simulink model "lane_rule"  (R2016b)
settings: Solver=VariableStepAuto  StartTime=0.0  StopTime=10.0  RelTol=1e-3
libraries: robotlib x13
settings Model: Creator=shota  LastModifiedBy=shota

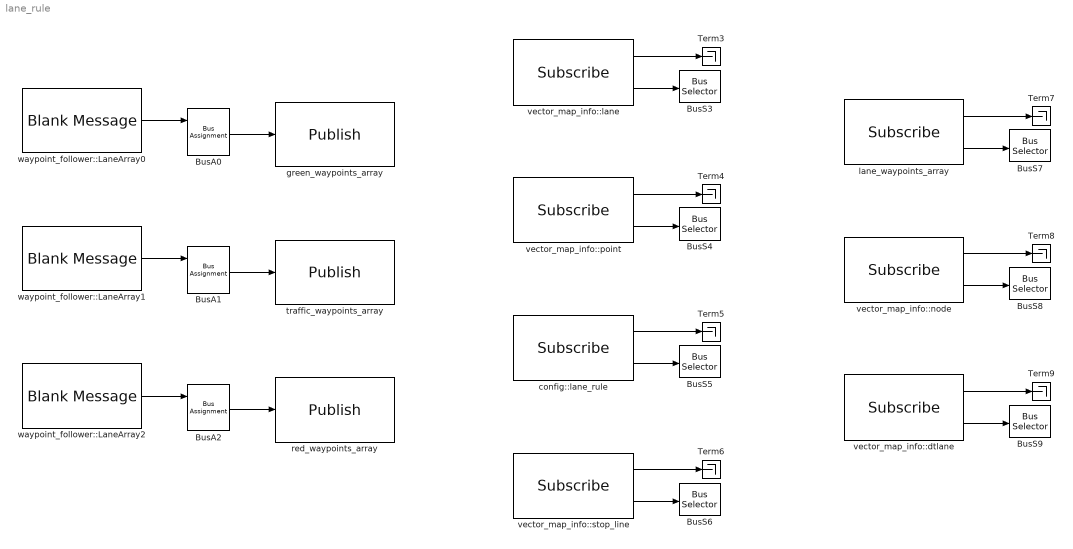
== system lane_rule ==
  BusA0 : BusAssignment  AssignedSignals=signal1
  BusA1 : BusAssignment  AssignedSignals=signal1
  BusA2 : BusAssignment  AssignedSignals=signal1
  BusS{3..9} (7 alike) : BusSelector  OutputSignals=signal1,signal2
  Term{3..9} (7 alike) : Terminator
  config::lane_rule : robotlib/Subscribe  SourceLibraryInfo=This block requires Robotics System Toolbox  topicSource=Specify your own  topic=/config/lane_rule  messageType=runtime_manager/ConfigLaneRule  sampleTime=-1  messageQueueLength=1
  green_waypoints_array : robotlib/Publish  SourceLibraryInfo=This block requires Robotics System Toolbox  topicSource=Specify your own  topic=/green_waypoints_array  messageType=waypoint_follower/LaneArray  messageQueueLength=1
  lane_waypoints_array : robotlib/Subscribe  SourceLibraryInfo=This block requires Robotics System Toolbox  topicSource=Specify your own  topic=/lane_waypoints_array  messageType=waypoint_follower/LaneArray  sampleTime=-1  messageQueueLength=1
  red_waypoints_array : robotlib/Publish  SourceLibraryInfo=This block requires Robotics System Toolbox  topicSource=Specify your own  topic=/red_waypoints_array  messageType=waypoint_follower/LaneArray  messageQueueLength=1
  traffic_waypoints_array : robotlib/Publish  SourceLibraryInfo=This block requires Robotics System Toolbox  topicSource=Specify your own  topic=/traffic_waypoints_array  messageType=waypoint_follower/LaneArray  messageQueueLength=1
  vector_map_info::dtlane : robotlib/Subscribe  SourceLibraryInfo=This block requires Robotics System Toolbox  topicSource=Specify your own  topic=/vector_map_info/dtlane  messageType=vector_map_msgs/DTLaneArray  sampleTime=-1  messageQueueLength=1
  vector_map_info::lane : robotlib/Subscribe  SourceLibraryInfo=This block requires Robotics System Toolbox  topicSource=Specify your own  topic=/vector_map_info/lane  messageType=vector_map_msgs/LaneArray  sampleTime=-1  messageQueueLength=1
  vector_map_info::node : robotlib/Subscribe  SourceLibraryInfo=This block requires Robotics System Toolbox  topicSource=Specify your own  topic=/vector_map_info/node  messageType=vector_map_msgs/NodeArray  sampleTime=-1  messageQueueLength=1
  vector_map_info::point : robotlib/Subscribe  SourceLibraryInfo=This block requires Robotics System Toolbox  topicSource=Specify your own  topic=/vector_map_info/point  messageType=vector_map_msgs/PointArray  sampleTime=-1  messageQueueLength=1
  vector_map_info::stop_line : robotlib/Subscribe  SourceLibraryInfo=This block requires Robotics System Toolbox  topicSource=Specify your own  topic=/vector_map_info/stop_line  messageType=vector_map_msgs/StopLineArray  sampleTime=-1  messageQueueLength=1
  waypoint_follower::LaneArray0 : robotlib/Blank Message  SourceLibraryInfo=This block requires Robotics System Toolbox  messageType=waypoint_follower/LaneArray  SampleTime=inf
  waypoint_follower::LaneArray1 : robotlib/Blank Message  SourceLibraryInfo=This block requires Robotics System Toolbox  messageType=waypoint_follower/LaneArray  SampleTime=inf
  waypoint_follower::LaneArray2 : robotlib/Blank Message  SourceLibraryInfo=This block requires Robotics System Toolbox  messageType=waypoint_follower/LaneArray  SampleTime=inf
  wires:
  waypoint_follower::LaneArray0/1 -> BusA0/1
  BusA0/1 -> green_waypoints_array/1
  waypoint_follower::LaneArray1/1 -> BusA1/1
  BusA1/1 -> traffic_waypoints_array/1
  waypoint_follower::LaneArray2/1 -> BusA2/1
  BusA2/1 -> red_waypoints_array/1
  vector_map_info::lane/1 -> Term3/1
  vector_map_info::lane/2 -> BusS3/1
  vector_map_info::point/1 -> Term4/1
  vector_map_info::point/2 -> BusS4/1
  config::lane_rule/1 -> Term5/1
  config::lane_rule/2 -> BusS5/1
  vector_map_info::stop_line/1 -> Term6/1
  vector_map_info::stop_line/2 -> BusS6/1
  lane_waypoints_array/1 -> Term7/1
  lane_waypoints_array/2 -> BusS7/1
  vector_map_info::node/1 -> Term8/1
  vector_map_info::node/2 -> BusS8/1
  vector_map_info::dtlane/1 -> Term9/1
  vector_map_info::dtlane/2 -> BusS9/1
